simulink model "sfcndemo_counter_cpp"  (Simulink 7.6)
settings: Solver=FixedStepDiscrete  StartTime=0.0  StopTime=9.9  FixedStep=1  RelTol=1e-3
Description:
  | Counter Implemented in a C++ S-function
settings Model: Creator=The MathWorks Inc.  ExtModeTrigMode=oneshot  ExtModeArmWhenConnect=off  ExtModeAutoUpdateStatusClock=off
settings DataIOCC: LimitDataPoints=off
settings OptimizationCC: BlockReduction=off  BooleanDataType=off  InlineInvariantSignals=on  InitFltsAndDblsToZero=on
settings DebuggingCC: SaveWithParameterizedLinksMsg=none  SignalResolutionControl=TryResolveAllWithWarning  SolverPrmCheckMsg=none  MultiTaskDSMMsg=warning  MultiTaskCondExecSysMsg=none
settings RTWCC: RetainRTWFile=on  ProcessScript=grt_make_rtw_hook  IncludeERTFirstTime=on
settings CodeAppCC: CustomSymbolStrFcn=$F$N$M
settings GRTTargetCC: TargetFcnLib=ansi_tfl_tmw.mat

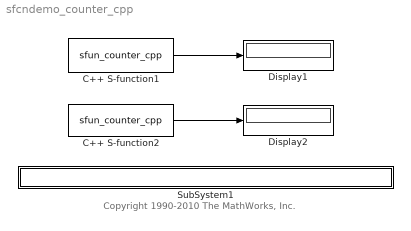
== system sfcndemo_counter_cpp ==
  note: Copyright 1990-2010 The MathWorks, Inc.
  C++ S-function1 : S-Function  FunctionName=sfun_counter_cpp  Parameters=1  EnableBusSupport=off
  C++ S-function2 : S-Function  FunctionName=sfun_counter_cpp  Parameters=2  EnableBusSupport=off
  Display1 : Display
  Display2 : Display
  SubSystem1 : Subsystem  mask{filename=sfun_counter_cpp.cpp}
      mask init:
      | x=sfundemo_maskdisp;
      settings: AttributesFormatString=\n  OpenFcn=sfundemo_openfcn
      mask Display: disp(x);
  wires:
  C++ S-function1/1 -> Display1/1
  C++ S-function2/1 -> Display2/1

== system sfcndemo_counter_cpp/SubSystem1 ==
